simulink model "dsa2k_iwave_rfi"  (R2021a)
settings: Solver=VariableStepAuto  StartTime=0.0  StopTime=10.0  RelTol=1e-3
undefined symbols (not defined in the file): datetime, i, posixtime
libraries: xbsIndex_r4 x3053, casper_library_misc x61, rtr_casper_dsp_lib x31, xps_library x1
(part 1 of 43)
settings Model: Creator=jackh  LastModifiedBy=jackh

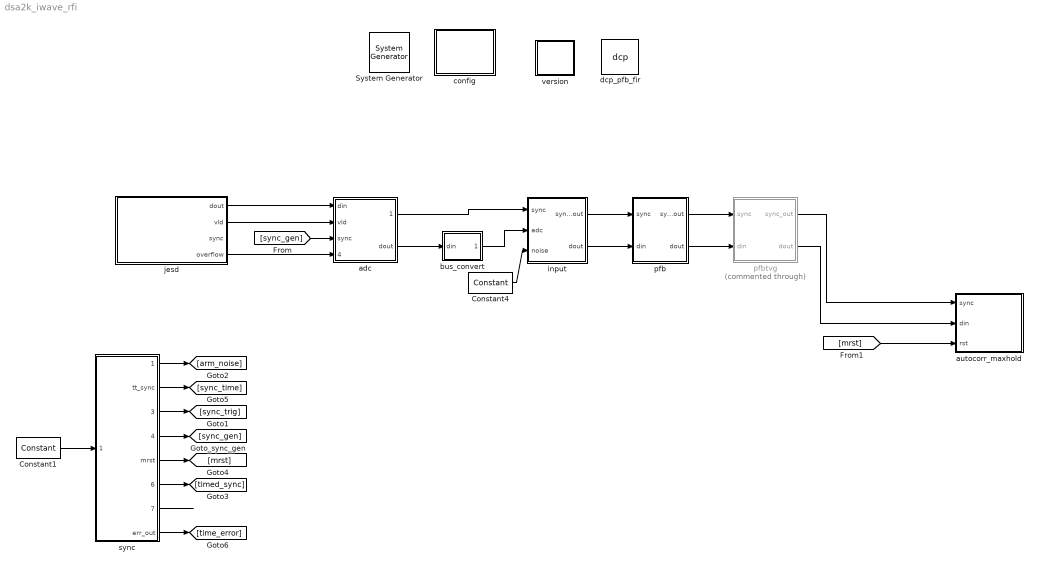
== system dsa2k_iwave_rfi ==
  " System Generator" : xbsIndex_r4/ System Generator  Tag=genX  xilinxfamily=zynquplus  part=xczu11eg  speed=-1-i  package=ffvc1760  synthesis_tool=XST  clock_wrapper=Clock Enables  directory=/home/jackh/src/dsa2000-fpga/firmware/src/models/dsa2k_iwave_rfi/sysgen  proj_type=Vivado  Synth_file=Vivado Synthesis Defaults  Impl_file=Vivado Implementation Defaults  testbench=off  simulink_period=1  sysclk_period=3.3333  dcm_input_clock_period=10  incr_netlist=off  trim_vbits=Everywhere in SubSystem  dbl_ovrd=According to Block Masks  core_generation=According to Block Masks  run_coregen=off  deprecated_control=off  eval_field=0  block_type=sysgen
  Constant1 : xbsIndex_r4/Constant  const=0  gui_display_data_type=Boolean  arith_type=Boolean  n_bits=16  bin_pt=14  preci_type=Single  exp_width=8  frac_width=24  explicit_period=on  period=1  equ=P=C  opselect=C  inp2=PCIN>>17  opr=+  inp1=P  carry=CIN  dbl_ovrd=off  block_type=constant
  Constant4 : xbsIndex_r4/Constant  const=0  gui_display_data_type=Fixed-point  arith_type=Unsigned  n_bits=12*32  bin_pt=0  preci_type=Single  exp_width=8  frac_width=24  explicit_period=on  period=1  equ=P=C  opselect=C  inp2=PCIN>>17  opr=+  inp1=P  carry=CIN  dbl_ovrd=off  block_type=constant
  adc : Subsystem  Tag=rtr:adc  AncestorBlock=rtr_casper_dsp_lib/adc  mask{ver_major=1, ver_minor=0, n_input=2, dtype='>i2'}
      mask prompts: ver_major "Block major version"; ver_minor "Block minor version"; n_input "Number of independent inputs"; dtype "Numpy sample data type"
  autocorr_maxhold : Subsystem  Tag=rtr:autocorr-maxhold  AncestorBlock=rtr_casper_dsp_lib/autocorr_maxhold  mask{rev_major=1, rev_minor=0, n_chan_serial_bits=14-3, n_chan_parallel_bits=3, n_input_serial_bits=0, n_input=2}
      mask prompts: rev_major "Major revision number"; rev_minor "Minor revision number"; n_chan_serial_bits "Number of *SERIAL* channels (2^?)"; n_chan_parallel_bits "Number of *PARALLEL* channels (2^?)"; n_input_serial_bits "Number of serial inputs (2^?)"; n_input "Total number of inputs"
  bus_convert : Subsystem  AncestorBlock=casper_library_bus/bus_convert  mask(bus_convert){n_bits_in=ones(32,1)*16, bin_pt_in=ones(32,1)*15, cmplx=off, n_bits_out=12, bin_pt_out=11, quantization=0, overflow=0, csp_latency=0, of=off, misc=off}
      mask prompts: n_bits_in "input bit widths"; bin_pt_in "input binary points"; cmplx "input complex"; n_bits_out "output bit widths"; bin_pt_out "output binary points"; quantization "quantization strategy (Truncate=0, Round  (unbiased: +/- Inf)=1, Round (unbiased: Even Values)=2)"; overflow "overflow strategy (Wrap=0, Saturate=1, Flag as error=2)"; csp_latency "latency"; of "overflow indication"; misc "misc support"
      mask help: Convert components of busses
      mask init:
      | bus_convert_init(gcb, ...
      |     'n_bits_in', n_bits_in, ...
      |     'bin_pt_in', bin_pt_in, ...
      |     'cmplx', cmplx, ...
      |     'n_bits_out', n_bits_out, ...
      |     'bin_pt_out', bin_pt_out, ...
      |     'quantization', quantization, ...
      |     'overflow', overflow, ...
      |     'csp_latency', csp_latency, ...
      |     'misc', misc, ...
      |     'of', of);
  config : Subsystem  Tag=xps:xsg  mask(xsg core config){hw_sys=iwave_zu11:xczu11eg, clk_src=adc_clk, clk_rate=4800/16, no_block_diagram=on, sample_period=1, synthesis_tool=XST}
      mask prompts: hw_sys "Hardware Platform"; clk_src "User IP Clock source"; clk_rate "User IP Clock Rate (MHz)"; no_block_diagram "Skip inclusion of infrastructure block diagram"; sample_period "Sample Period"; synthesis_tool "Synthesis Tool:"
      mask help:
      | The XSG Core Config block is used to configure the System Generator design
      | for the casper_xps toolflow. Settings here are used to configure the
      | Xilinx System Generator block parameters automatically, and control toolflow
      | script  execution. It needs to be at the top level of all designs being compiled
      | with the casper_xps toolflow.
      mask init:
      | xps_xsg_iwave_zu11_conf_mask;
      mask Help: eval('xlWeb([getenv(''MLIB_ROOT''), ''\doc\html\sys_xsg_core_config\sys_xsg_core_config.html''])')
      mask TypeOptions hw_sys: iwave_zu11:xczu11eg
      mask TypeOptions clk_src: sys_clk | adc_clk | clk300mhz
      mask TypeOptions synthesis_tool: Leonardo Spectrum | Synplify | Synplify Pro | XST
      mask Display: fprintf(['iWave_ZU11']);
  dcp_pfb_fir : xps_library/Utilities/dcp  Tag=xps:dcp  dcp_file=[fileparts(which(bdroot)) '/dsp/pfb_2p_32kpt_12i_18o_core/pfb_2p_32kpt_12i_18o_core.dcp']
      settings: SourceProductName=CASPER XPS Blockset
  input : Subsystem  Tag=rtr:input  AncestorBlock=rtr_casper_dsp_lib/input  mask{rev_major=1, rev_minor=0, n_bits=12, n_parallel=16, n_inputs=2}
      mask prompts: rev_major "Major revision number"; rev_minor "Minor revision number"; n_bits "Number of bits per samples"; n_parallel "Parallel Samples per input"; n_inputs "Parallel inputs"
  jesd : Subsystem  Tag=xps:adi_jesd  mask(xsg_adi_jesd){fmc_port=0, adi_ip_path=/home/jackh/src/dsa2000-fpga/firmware/lib/adi_hdl/library, sample_rate_mhz=4800}
      mask prompts: fmc_port "FMC Port Number"; adi_ip_path "Path to ADI IP repository"; sample_rate_mhz "Sample rate (Msps)"
      mask init:
      | adi_jesd_init()
      mask Help: eval('xlWeb([getenv(''MLIB_ROOT''), ''\doc\html\sys_xsg_core_config\sys_xsg_core_config.html''])')
  pfb : Subsystem  Tag=rtr:pfb  AncestorBlock=rtr_casper_dsp_lib/pfb  mask{rev_major=1, rev_minor=0, fft_bits=15}
      mask prompts: rev_major "Major revision number"; rev_minor "Minor revision number"; fft_bits "FFT length (2^?)"
  pfbtvg : Subsystem  Commented=through  mask{serial_chan_bits=14-3}
      mask prompts: serial_chan_bits "Serial channels (2^?)"
  sync : Subsystem  Tag=rtr:sync  AncestorBlock=rtr_casper_dsp_lib/sync  mask{rev_major=1, rev_minor=0, sync_lsb_bits=14, sync_period=12800000}
      mask prompts: rev_major "Rev Major"; rev_minor "Rev Minor"; sync_lsb_bits "Allowed sync granularity (2^?)"; sync_period "Expected_sync_period"
  version : Subsystem  Tag=rtr:version  AncestorBlock=rtr_casper_dsp_lib/version  mask{rev_major=1, rev_minor=0, fw_type=9, fw_ver_maj=1, fw_ver_min=0, fw_ver_rev=0, fw_ver_bugfix=0}
      mask prompts: rev_major "Rev Major (this block, not the firmware!)"; rev_minor "Rev Minor (this block, not the firmware!)"; fw_type "Firmware Type"; fw_ver_maj "Major version"; fw_ver_min "Minor version"; fw_ver_rev "Revision"; fw_ver_bugfix "Bugfix"
  wires:
  sync/1(arm_noise) -> [arm_noise]
  sync/2(tt_sync) -> [sync_time]
  sync/5(mrst) -> [mrst]
  sync/3(ext_sync) -> [sync_trig]
  sync/6(timed_sync) -> [timed_sync]
  sync/4(sync_out) -> [sync_gen]
  sync/8(err_out) -> [time_error]
  sync/7(tt_int_out) -> ?
  Constant1/1 -> sync/1(sync_in)
  adc/2(dout) -> bus_convert/1(din)
  pfbtvg/1(sync_out) -> autocorr_maxhold/1(sync)
  [mrst] -> autocorr_maxhold/3(rst)
  jesd/2(vld) -> adc/2(vld)
  jesd/4(overflow) -> adc/4(overflow)
  jesd/1(dout) -> adc/1(din)
  pfbtvg/2(dout) -> autocorr_maxhold/2(din)
  pfb/1(sync_out) -> pfbtvg/1(sync)
  pfb/2(dout) -> pfbtvg/2(din)
  [sync_gen] -> adc/3(sync)
  Constant4/1 -> input/3(noise)
  input/1(sync_out) -> pfb/1(sync)
  bus_convert/1(dout) -> input/2(adc)
  adc/1(sync_out) -> input/1(sync)
  input/2(dout) -> pfb/2(din)

== system dsa2k_iwave_rfi/adc ==
  din : Inport
  vld : Inport  Port=2
  sync : Inport  Port=3
  overflow : Inport  Port=4
  Inverter1 : xbsIndex_r4/Inverter  en=off  latency=1  dbl_ovrd=off  block_type=inv
  Logical : xbsIndex_r4/Logical  logical_function=OR  inputs=2  en=off  latency=0  precision=Full  arith_type=Unsigned  n_bits=16  bin_pt=0  align_bp=on  dbl_ovrd=off  block_type=logical
  Scope2 : Scope
  Scope3 : Scope
  Scope4 : Scope
  bitflip : Subsystem
  block_info : Subsystem  AncestorBlock=rtr_casper_dsp_lib/block_info
      mask init:
      | parent = get_param(gcb, 'Parent');
      | try
      |     params = get_param(parent, 'DialogParameters');
      | catch
      |     params = {};
      | end
      | info.library = 'rtr';
      | info.block_type = get_param(parent, 'Tag');
      | info.block_name = parent;
      | 
      | if length(params) > 0
      |     param_names = fieldnames(params);
      | else
      |     param_names = {};
      | end
      | n_param = length(param_names);
      | 
      | for n = 1:n_param
      |     param = param_names{n};
      |     val = get_param(parent, param);
      |     try
      |         val = eval(val);
      |     catch
      |     end
      |     info = setfield(info, param, val);
      | end
      | 
      | munge_block(gcb);
      | set_param([gcb '/info'], 'info', jsonencode(info));
  counter_led3 : xbsIndex_r4/Counter  cnt_type=Free Running  cnt_to=Inf  operation=Up  start_count=0  cnt_by_val=1  arith_type=Unsigned  n_bits=32  bin_pt=0  load_pin=off  rst=off  en=on  explicit_period=on  period=1  use_behavioral_HDL=off  implementation=Fabric  dbl_ovrd=off  block_type=counter
  counter_led4 : xbsIndex_r4/Counter  cnt_type=Free Running  cnt_to=Inf  operation=Up  start_count=0  cnt_by_val=1  arith_type=Unsigned  n_bits=32  bin_pt=0  load_pin=off  rst=off  en=on  explicit_period=on  period=1  use_behavioral_HDL=off  implementation=Fabric  dbl_ovrd=off  block_type=counter
  counter_led5 : xbsIndex_r4/Counter  cnt_type=Free Running  cnt_to=Inf  operation=Up  start_count=0  cnt_by_val=1  arith_type=Unsigned  n_bits=32  bin_pt=0  load_pin=off  rst=off  en=on  explicit_period=on  period=1  use_behavioral_HDL=off  implementation=Fabric  dbl_ovrd=off  block_type=counter
  edge_detect : casper_library_misc/edge_detect  edge=Rising  polarity=Active High  x_in=[0 0.08 0.08 0.16 0.16 0.24 0.24 0.32 0.32 0.4]  y_in="[-1 -1  1  1  1  1  1  1  1  1]"  x_out=[0.6 0.68 0.68 0.76 0.76 0.84 0.84 0.92 0.92 1]  y_out="[-1 -1  1  1 -1 -1 -1 -1 -1 -1]"
  edge_detect1 : casper_library_misc/edge_detect  edge=Rising  polarity=Active High  x_in=[0 0.08 0.08 0.16 0.16 0.24 0.24 0.32 0.32 0.4]  y_in="[-1 -1  1  1  1  1  1  1  1  1]"  x_out=[0.6 0.68 0.68 0.76 0.76 0.84 0.84 0.92 0.92 1]  y_out="[-1 -1  1  1 -1 -1 -1 -1 -1 -1]"
  invalid_counter : Subsystem  Tag=xps:sw_reg  AncestorBlock=xps_library/Memory/software_register  mask(swreg){io_dir=To Processor, io_delay=0, init_val=0, sample_period=1, names=reg, bitwidths=32, bin_pts=0, arith_types=0, sim_port=on, show_format=off}
      mask prompts: io_dir "I/O direction"; io_delay "I/O delay"; init_val "Initial Value"; sample_period "Sample period"; names "Bitfield names [msb...lsb]"; bitwidths "Bitfield widths"; bin_pts "Bitfield binary pts"; arith_types "Bitfield types, ufix=0, fix=1, bool=2"; sim_port "Provide sim input/output?"; show_format "Print format string?"
      mask help: A 32-bit software-accessible register. Can be divided into bitfields of varying widths and types using the fields in the block mask.
      mask init:
      | swreg_init(gcb)
      settings: AttributesFormatString=1output
      mask TypeOptions io_dir: To Processor | From Processor
      mask Callback io_dir:
      | mask_enables = get_param(gcb, 'MaskEnables');
      | mask_names = get_param(gcb, 'MaskNames');
      | if strcmp(get_param(gcb, 'io_dir'), 'To Processor'),
      |     mask_enables{ismember(mask_names, 'sample_period')} = 'off';
      | else
      |     mask_enables{ismember(mask_names, 'sample_period')} = 'on';
      | end
      | set_param(gcb, 'MaskEnables', mask_enables);
      mask DialogControl ParameterTabVar0 Prompt: Setup
  overflow_counter : Subsystem  Tag=xps:sw_reg  AncestorBlock=xps_library/Memory/software_register  mask(swreg){io_dir=To Processor, io_delay=0, init_val=0, sample_period=1, names=reg, bitwidths=32, bin_pts=0, arith_types=0, sim_port=on, show_format=off}
      mask prompts: io_dir "I/O direction"; io_delay "I/O delay"; init_val "Initial Value"; sample_period "Sample period"; names "Bitfield names [msb...lsb]"; bitwidths "Bitfield widths"; bin_pts "Bitfield binary pts"; arith_types "Bitfield types, ufix=0, fix=1, bool=2"; sim_port "Provide sim input/output?"; show_format "Print format string?"
      mask help: A 32-bit software-accessible register. Can be divided into bitfields of varying widths and types using the fields in the block mask.
      mask init:
      | swreg_init(gcb)
      settings: AttributesFormatString=1output
      mask TypeOptions io_dir: To Processor | From Processor
      mask Callback io_dir:
      | mask_enables = get_param(gcb, 'MaskEnables');
      | mask_names = get_param(gcb, 'MaskNames');
      | if strcmp(get_param(gcb, 'io_dir'), 'To Processor'),
      |     mask_enables{ismember(mask_names, 'sample_period')} = 'off';
      | else
      |     mask_enables{ismember(mask_names, 'sample_period')} = 'on';
      | end
      | set_param(gcb, 'MaskEnables', mask_enables);
      mask DialogControl ParameterTabVar0 Prompt: Setup
  snapshot_arm : Subsystem  Tag=xps:sw_reg  AncestorBlock=xps_library/Memory/software_register  mask(swreg){io_dir=From Processor, io_delay=0, init_val=0, sample_period=1, names=reg, bitwidths=1, bin_pts=0, arith_types=2, sim_port=on, show_format=off}
      mask prompts: io_dir "I/O direction"; io_delay "I/O delay"; init_val "Initial Value"; sample_period "Sample period"; names "Bitfield names [msb...lsb]"; bitwidths "Bitfield widths"; bin_pts "Bitfield binary pts"; arith_types "Bitfield types, ufix=0, fix=1, bool=2"; sim_port "Provide sim input/output?"; show_format "Print format string?"
      mask help: A 32-bit software-accessible register. Can be divided into bitfields of varying widths and types using the fields in the block mask.
      mask init:
      | swreg_init(gcb)
      settings: AttributesFormatString=1input
      mask TypeOptions io_dir: To Processor | From Processor
      mask Callback io_dir:
      | mask_enables = get_param(gcb, 'MaskEnables');
      | mask_names = get_param(gcb, 'MaskNames');
      | if strcmp(get_param(gcb, 'io_dir'), 'To Processor'),
      |     mask_enables{ismember(mask_names, 'sample_period')} = 'off';
      | else
      |     mask_enables{ismember(mask_names, 'sample_period')} = 'on';
      | end
      | set_param(gcb, 'MaskEnables', mask_enables);
      mask DialogControl ParameterTabVar0 Prompt: Setup
  snapshot_trig : Subsystem  Tag=xps:sw_reg  AncestorBlock=xps_library/Memory/software_register  mask(swreg){io_dir=From Processor, io_delay=0, init_val=0, sample_period=1, names=reg, bitwidths=1, bin_pts=0, arith_types=2, sim_port=on, show_format=off}
      mask prompts: io_dir "I/O direction"; io_delay "I/O delay"; init_val "Initial Value"; sample_period "Sample period"; names "Bitfield names [msb...lsb]"; bitwidths "Bitfield widths"; bin_pts "Bitfield binary pts"; arith_types "Bitfield types, ufix=0, fix=1, bool=2"; sim_port "Provide sim input/output?"; show_format "Print format string?"
      mask help: A 32-bit software-accessible register. Can be divided into bitfields of varying widths and types using the fields in the block mask.
      mask init:
      | swreg_init(gcb)
      settings: AttributesFormatString=1input
      mask TypeOptions io_dir: To Processor | From Processor
      mask Callback io_dir:
      | mask_enables = get_param(gcb, 'MaskEnables');
      | mask_names = get_param(gcb, 'MaskNames');
      | if strcmp(get_param(gcb, 'io_dir'), 'To Processor'),
      |     mask_enables{ismember(mask_names, 'sample_period')} = 'off';
      | else
      |     mask_enables{ismember(mask_names, 'sample_period')} = 'on';
      | end
      | set_param(gcb, 'MaskEnables', mask_enables);
      mask DialogControl ParameterTabVar0 Prompt: Setup
  ss : Subsystem
  sync_counter : Subsystem  Tag=xps:sw_reg  AncestorBlock=xps_library/Memory/software_register  mask(swreg){io_dir=To Processor, io_delay=0, init_val=0, sample_period=1, names=reg, bitwidths=32, bin_pts=0, arith_types=0, sim_port=on, show_format=off}
      mask prompts: io_dir "I/O direction"; io_delay "I/O delay"; init_val "Initial Value"; sample_period "Sample period"; names "Bitfield names [msb...lsb]"; bitwidths "Bitfield widths"; bin_pts "Bitfield binary pts"; arith_types "Bitfield types, ufix=0, fix=1, bool=2"; sim_port "Provide sim input/output?"; show_format "Print format string?"
      mask help: A 32-bit software-accessible register. Can be divided into bitfields of varying widths and types using the fields in the block mask.
      mask init:
      | swreg_init(gcb)
      settings: AttributesFormatString=1output
      mask TypeOptions io_dir: To Processor | From Processor
      mask Callback io_dir:
      | mask_enables = get_param(gcb, 'MaskEnables');
      | mask_names = get_param(gcb, 'MaskNames');
      | if strcmp(get_param(gcb, 'io_dir'), 'To Processor'),
      |     mask_enables{ismember(mask_names, 'sample_period')} = 'off';
      | else
      |     mask_enables{ismember(mask_names, 'sample_period')} = 'on';
      | end
      | set_param(gcb, 'MaskEnables', mask_enables);
      mask DialogControl ParameterTabVar0 Prompt: Setup
  sync_out : Outport
  dout : Outport  Port=2
  wires:
  Logical/1 -> ss/2(trig)
  Inverter1/1 -> counter_led5/1
  invalid_counter/1(sim_out_reg) -> Scope4/1
  counter_led5/1 -> invalid_counter/1(out_reg)
  vld/1 -> Inverter1/1, ss/1(we)
  counter_led4/1 -> sync_counter/1(out_reg)
  sync/1 -> Logical/1, counter_led4/1, sync_out/1
  edge_detect1/1 -> Logical/2
  sync_counter/1(sim_out_reg) -> Scope3/1
  snapshot_trig/1(in_reg) -> edge_detect1/1
  snapshot_arm/1(in_reg) -> edge_detect/1
  edge_detect/1 -> ss/3(arm)
  overflow_counter/1(sim_out_reg) -> Scope2/1
  counter_led3/1 -> overflow_counter/1(out_reg)
  overflow/1 -> counter_led3/1
  din/1 -> bitflip/1(bus_in)
  bitflip/1(bus_out) -> ss/4(bus_in), dout/1

== system dsa2k_iwave_rfi/autocorr_maxhold ==
  note: acc_len in spectra
  sync : Inport
  din : Inport  Port=2
  rst : Inport  Port=3
  0 : Subsystem  mask{nchan_bits=n_chan_serial_bits, npol_bits=n_input_serial_bits}
      mask prompts: nchan_bits "Number of channels (2^?)"; npol_bits "Number of pols (2^?)"
  1 : Subsystem  mask{nchan_bits=n_chan_serial_bits, npol_bits=n_input_serial_bits}
      mask prompts: nchan_bits "Number of channels (2^?)"; npol_bits "Number of pols (2^?)"
  Constant6 : Constant  Value=1024
  Counter1 : xbsIndex_r4/Counter  cnt_type=Free Running  cnt_to=Inf  operation=Up  start_count=0  cnt_by_val=1  arith_type=Unsigned  n_bits=32  bin_pt=0  load_pin=off  rst=off  en=on  explicit_period=on  period=1  use_behavioral_HDL=on  implementation=Fabric  dbl_ovrd=off  block_type=counter
  Delay1 : xbsIndex_r4/Delay  rst=off  infoeditControl=Selection of Reset will increase slice count due to use of real FFs and instead of SRLs  en=off  latency=1  reg_retiming=off  dbl_ovrd=off  block_type=delay
  Delay2 : xbsIndex_r4/Delay  rst=off  infoeditControl=Selection of Reset will increase slice count due to use of real FFs and instead of SRLs  en=off  latency=1  reg_retiming=on  dbl_ovrd=off  block_type=delay
  Slice1 : xbsIndex_r4/Slice  nbits=32 - n_chan_serial_bits - n_input_serial_bits  boolean_output=off  mode=Lower Bit Location + Width  bit1=0  base1=MSB of Input  bit0=0  base0=LSB of Input  dbl_ovrd=off  block_type=slice
  acc_cnt : Subsystem  Tag=xps:sw_reg  AncestorBlock=xps_library/Memory/software_register  mask(swreg){io_dir=To Processor, io_delay=0, init_val=0, sample_period=1, names=reg, bitwidths=32, bin_pts=0, arith_types=0, sim_port=on, show_format=on, desc_str=|}
      mask desc_str=|
      | 32-bit wrapping accumulation counter, which increments each
      | time a new accumulation is recorded to RAM.
      | There is no buffer locking when correlation data are
      | read, so this counter can be used to ensure that data
      | have not changed during a read.
      mask prompts: io_dir "I/O direction"; io_delay "I/O delay"; init_val "Initial Value"; sample_period "Sample period"; names "Bitfield names [msb...lsb]"; bitwidths "Bitfield widths"; bin_pts "Bitfield binary pts"; arith_types "Bitfield types, ufix=0, fix=1, bool=2"; sim_port "Provide sim input/output?"; show_format "Print format string?"; desc_str "Description"
      mask help: A 32-bit software-accessible register. Can be divided into bitfields of varying widths and types using the fields in the block mask.
      mask init:
      | swreg_init(gcb)
      settings: AttributesFormatString=1output:uf32.0 = 32 bits
      mask TypeOptions io_dir: To Processor | From Processor
      mask Callback io_dir:
      | mask_enables = get_param(gcb, 'MaskEnables');
      | mask_names = get_param(gcb, 'MaskNames');
      | if strcmp(get_param(gcb, 'io_dir'), 'To Processor'),
      |     mask_enables{ismember(mask_names, 'sample_period')} = 'off';
      | else
      |     mask_enables{ismember(mask_names, 'sample_period')} = 'on';
      | end
      | set_param(gcb, 'MaskEnables', mask_enables);
      mask DialogControl ParameterTabVar0 Prompt: Setup
  acc_len : Subsystem  Tag=xps:sw_reg  AncestorBlock=xps_library/Memory/software_register  mask(swreg){io_dir=From Processor, io_delay=0, init_val=0, sample_period=1, names=reg, bitwidths=32, bin_pts=0, arith_types=0, sim_port=on, show_format=on, desc_str=Accumulation length, in spectra.}
      mask prompts: io_dir "I/O direction"; io_delay "I/O delay"; init_val "Initial Value"; sample_period "Sample period"; names "Bitfield names [msb...lsb]"; bitwidths "Bitfield widths"; bin_pts "Bitfield binary pts"; arith_types "Bitfield types, ufix=0, fix=1, bool=2"; sim_port "Provide sim input/output?"; show_format "Print format string?"; desc_str "Description"
      mask help: A 32-bit software-accessible register. Can be divided into bitfields of varying widths and types using the fields in the block mask.
      mask init:
      | swreg_init(gcb)
      settings: AttributesFormatString=1input:uf32.0 = 32 bits
      mask TypeOptions io_dir: To Processor | From Processor
      mask Callback io_dir:
      | mask_enables = get_param(gcb, 'MaskEnables');
      | mask_names = get_param(gcb, 'MaskNames');
      | if strcmp(get_param(gcb, 'io_dir'), 'To Processor'),
      |     mask_enables{ismember(mask_names, 'sample_period')} = 'off';
      | else
      |     mask_enables{ismember(mask_names, 'sample_period')} = 'on';
      | end
      | set_param(gcb, 'MaskEnables', mask_enables);
      mask DialogControl ParameterTabVar0 Prompt: Setup
  block_info : Subsystem  AncestorBlock=rtr_casper_dsp_lib/block_info
      mask init: same as dsa2k_iwave_rfi/adc/block_info
  bus_expand : Subsystem  AncestorBlock=casper_library_flow_control/bus_expand  mask(bus_expand){mode=divisions of equal size, outputNum=2, outputWidth=36*8, outputBinaryPt=0, outputArithmeticType=0, show_format=off, outputToWorkspace=off, variablePrefix=out, outputToModelAsWell=on}
      mask prompts: outputNum "Number of outputs:"; outputWidth "Output width:"; outputBinaryPt "Output binary point position:"; outputArithmeticType "Output arithmetic type (ufix=0, fix=1, bool=2):"; show_format "Print format string?"; outputToWorkspace "Output to workspace?"; variablePrefix "Variable name prefix:"; outputToModelAsWell "Output to model as well?"
      mask help:
      | Expands a 'bus' made using a bus_create or Xilinx
      | concat block.
      | The input will be divided into the specified number
      | of outputs with the specified arithmetic types.
      | Divisions are made from most significant bit.
      mask init:
      | bus_expand_init(gcb,...
      |     'mode', mode, ...
      |     'outputNum', outputNum, ...
      |     'outputWidth', outputWidth, ...
      |     'outputBinaryPt', outputBinaryPt, ...
      |     'outputArithmeticType', outputArithmeticType, ...
      |     'show_format', show_format, ...
      |     'outputToWorkspace', outputToWorkspace, ...
      |     'variablePrefix', variablePrefix, ...
      |     'outputToModelAsWell', outputToModelAsWell);
      settings: AttributesFormatString=2 outputs
      mask TypeOptions mode: divisions of equal size | divisions of arbitrary size
      mask Callback mode: %bus_expand_callback();
      mask Callback outputWidth: %bus_expand_callback();
      mask Callback outputToWorkspace: %bus_expand_callback();
  trig : Subsystem  Tag=xps:sw_reg  AncestorBlock=xps_library/Memory/software_register  mask(swreg){io_dir=From Processor, io_delay=0, init_val=0, sample_period=1, names=reg, bitwidths=1, bin_pts=0, arith_types=2, sim_port=on, show_format=on, desc_str="Transition bit 0 from 0 to 1 to trigger a capture of the next valid accumulation"}
      mask prompts: io_dir "I/O direction"; io_delay "I/O delay"; init_val "Initial Value"; sample_period "Sample period"; names "Bitfield names [msb...lsb]"; bitwidths "Bitfield widths"; bin_pts "Bitfield binary pts"; arith_types "Bitfield types, ufix=0, fix=1, bool=2"; sim_port "Provide sim input/output?"; show_format "Print format string?"; desc_str "Description"
      mask help: A 32-bit software-accessible register. Can be divided into bitfields of varying widths and types using the fields in the block mask.
      mask init:
      | swreg_init(gcb)
      settings: AttributesFormatString=1input:b = 1 bits
      mask TypeOptions io_dir: To Processor | From Processor
      mask Callback io_dir:
      | mask_enables = get_param(gcb, 'MaskEnables');
      | mask_names = get_param(gcb, 'MaskNames');
      | if strcmp(get_param(gcb, 'io_dir'), 'To Processor'),
      |     mask_enables{ismember(mask_names, 'sample_period')} = 'off';
      | else
      |     mask_enables{ismember(mask_names, 'sample_period')} = 'on';
      | end
      | set_param(gcb, 'MaskEnables', mask_enables);
      mask DialogControl ParameterTabVar0 Prompt: Setup
  wires:
  Delay1/1 -> Counter1/1
  0/1(new_acc) -> [new_acc]
  [trig] -> 0/5(trig)
  trig/1(in_reg) -> [trig]
  [input0] -> 0/2(din)
  [acc_len] -> 0/4(acc_len)
  Counter1/1 -> Delay2/1
  Delay2/1 -> acc_cnt/1(out_reg)
  [new_acc] -> Delay1/1
  Slice1/1 -> [acc_len]
  Constant6/1 -> acc_len/1(sim_1)
  acc_len/1(in_reg) -> Slice1/1
  [rst] -> 0/3(rst)
  [sync] -> 0/1(sync)
  rst/1 -> [rst]
  sync/1 -> [sync]
  din/1 -> bus_expand/1(bus_in)
  bus_expand/1(msb_out2) -> [input0]
  bus_expand/2(lsb_out1) -> [input1]
  [sync] -> 1/1(sync)
  [rst] -> 1/3(rst)
  [acc_len] -> 1/4(acc_len)
  [input1] -> 1/2(din)
  [trig] -> 1/5(trig)

== system dsa2k_iwave_rfi/bus_convert ==
  din : Inport
  bussify : Subsystem  AncestorBlock=casper_library_flow_control/bus_create  mask(bus_create){inputNum=32}
      mask prompts: inputNum "Number of inputs:"
      mask init:
      | bus_create_init(gcb,...
      |     'inputNum', inputNum);
  conv{1..32} (32 alike) : xbsIndex_r4/Convert  gui_display_data_type=Fixed-point  arith_type="Signed  (2's comp)"  n_bits=12  bin_pt=11  float_type=Single  exp_bits=8  fraction_bits=24  quantization=Truncate  overflow=Wrap  en=off  latency=0  pipeline=on  dbl_ovrd=off  block_type=convert
  debus : Subsystem  AncestorBlock=casper_library_flow_control/bus_expand  mask(bus_expand){mode=divisions of arbitrary size, outputNum=2, outputWidth=[16;16;16;16;16;16;16;16;16;16;16;16;16;16;16;16;16;16;16;16;16;16;16;16;16;16;16;16;16;16;16;16], outputBinaryPt=[15;15;15;15;15;15;15;15;15;15;15;15;15;15;15;15;15;15;15;15;15;15;15;15;15;15;15;15;15;15;15;15], outputArithmeticType=[1 1 1 1 1 1 1 1 1 1 1 1 1 1 1 1 1 1 1 1 1 1 1 1 1 1 1 1 1 1 1 1], show_format=on, outputToWorkspace=off, variablePrefix=, outputToModelAsWell=on}
      mask prompts: outputNum "Number of outputs:"; outputWidth "Output width:"; outputBinaryPt "Output binary point position:"; outputArithmeticType "Output arithmetic type (ufix=0, fix=1, bool=2):"; show_format "Print format string?"; outputToWorkspace "Output to workspace?"; variablePrefix "Variable name prefix:"; outputToModelAsWell "Output to model as well?"
      mask help:
      | Expands a 'bus' made using a bus_create or Xilinx
      | concat block.
      | The input will be divided into the specified number
      | of outputs with the specified arithmetic types.
      | Divisions are made from most significant bit.
      mask init: same as dsa2k_iwave_rfi/autocorr_maxhold/bus_expand
      settings: AttributesFormatString=32 outputs: f16.15,f16.15,f16.15,f16.15,f16.15,f16.15,f16.15,f16.15,f16.15,f16.15,f16.15,f16.15,f16.15,f16.15,f16.15,f16.15,f16.15,f16.15,f16.15,f16.15,f16.15,f16.15,f16.15,f16.15,f16.15,f16.15,f16.15,f16.15,f16.15,f16.15,f16.15,f16.15,
      mask TypeOptions mode: divisions of equal size | divisions of arbitrary size
      mask Callback mode: %bus_expand_callback();
      mask Callback outputWidth: %bus_expand_callback();
      mask Callback outputToWorkspace: %bus_expand_callback();
  dout : Outport
  wires:
  din/1 -> debus/1(bus_in)
  debus/1(msb_out32) -> conv1/1
  debus/2(out31) -> conv2/1
  debus/3(out30) -> conv3/1
  debus/4(out29) -> conv4/1
  debus/5(out28) -> conv5/1
  debus/6(out27) -> conv6/1
  debus/7(out26) -> conv7/1
  debus/8(out25) -> conv8/1
  debus/9(out24) -> conv9/1
  debus/10(out23) -> conv10/1
  debus/11(out22) -> conv11/1
  debus/12(out21) -> conv12/1
  debus/13(out20) -> conv13/1
  debus/14(out19) -> conv14/1
  debus/15(out18) -> conv15/1
  debus/16(out17) -> conv16/1
  debus/17(out16) -> conv17/1
  debus/18(out15) -> conv18/1
  debus/19(out14) -> conv19/1
  debus/20(out13) -> conv20/1
  debus/21(out12) -> conv21/1
  debus/22(out11) -> conv22/1
  debus/23(out10) -> conv23/1
  debus/24(out9) -> conv24/1
  debus/25(out8) -> conv25/1
  debus/26(out7) -> conv26/1
  debus/27(out6) -> conv27/1
  debus/28(out5) -> conv28/1
  debus/29(out4) -> conv29/1
  debus/30(out3) -> conv30/1
  debus/31(out2) -> conv31/1
  debus/32(lsb_out1) -> conv32/1
  conv1/1 -> bussify/1(in1)
  conv2/1 -> bussify/2(in2)
  conv3/1 -> bussify/3(in3)
  conv4/1 -> bussify/4(in4)
  conv5/1 -> bussify/5(in5)
  conv6/1 -> bussify/6(in6)
  conv7/1 -> bussify/7(in7)
  conv8/1 -> bussify/8(in8)
  conv9/1 -> bussify/9(in9)
  conv10/1 -> bussify/10(in10)
  conv11/1 -> bussify/11(in11)
  conv12/1 -> bussify/12(in12)
  conv13/1 -> bussify/13(in13)
  conv14/1 -> bussify/14(in14)
  conv15/1 -> bussify/15(in15)
  conv16/1 -> bussify/16(in16)
  conv17/1 -> bussify/17(in17)
  conv18/1 -> bussify/18(in18)
  conv19/1 -> bussify/19(in19)
  conv20/1 -> bussify/20(in20)
  conv21/1 -> bussify/21(in21)
  conv22/1 -> bussify/22(in22)
  conv23/1 -> bussify/23(in23)
  conv24/1 -> bussify/24(in24)
  conv25/1 -> bussify/25(in25)
  conv26/1 -> bussify/26(in26)
  conv27/1 -> bussify/27(in27)
  conv28/1 -> bussify/28(in28)
  conv29/1 -> bussify/29(in29)
  conv30/1 -> bussify/30(in30)
  conv31/1 -> bussify/31(in31)
  conv32/1 -> bussify/32(in32)
  bussify/1(bus_out) -> dout/1

== system dsa2k_iwave_rfi/config ==

== system dsa2k_iwave_rfi/input ==
  sync : Inport
  adc : Inport  Port=2
  noise : Inport  Port=3
  Constant4 : xbsIndex_r4/Constant  const=0  gui_display_data_type=Fixed-point  arith_type=Unsigned  n_bits=n_bits * n_parallel * n_inputs  bin_pt=0  preci_type=Single  exp_width=8  frac_width=24  explicit_period=on  period=1  equ=P=C  opselect=C  inp2=PCIN>>17  opr=+  inp1=P  carry=CIN  dbl_ovrd=off  block_type=constant
  bit_stats : Subsystem  Commented=on
  block_info : Subsystem  AncestorBlock=rtr_casper_dsp_lib/block_info
      mask init: same as dsa2k_iwave_rfi/adc/block_info
  bus_mux1 : Subsystem  AncestorBlock=casper_library_bus/bus_mux  mask(bus_mux){n_inputs=3, n_bits=n_bits * n_parallel * ones(n_inputs,1), cmplx=off, misc=on, mux_latency=1}
      mask prompts: n_inputs "number of inputs"; n_bits "input bit widths"; cmplx "complex data"; misc "misc support"; mux_latency "mux latency"
      mask help: Mux components of bus
      mask init:
      | bus_mux_init(gcb, ...
      |     'n_inputs', n_inputs, ...
      |     'n_bits', n_bits, ...
      |     'cmplx', cmplx, ...
      |     'misc', misc, ...
      |     'mux_latency', mux_latency);
  rms : Subsystem
  slice3 : xbsIndex_r4/Slice  nbits=2*2  boolean_output=off  mode=Upper Bit Location + Width  bit1=0  base1=MSB of Input  bit0=0  base0=LSB of Input  dbl_ovrd=off  block_type=slice
  source_sel0 : Subsystem  Tag=xps:sw_reg  AncestorBlock=xps_library/Memory/software_register  mask(swreg){io_dir=From Processor, io_delay=0, init_val=0, sample_period=1, names=reg, bitwidths=32, bin_pts=0, arith_types=0, sim_port=on, show_format=off, desc_str=|}
      mask desc_str=|
      | Selector control to determine if signal streams carry
      | ADC samples, digital noise samples, or zeros.
      | Streams ``n=0..15`` is controlled by register
      | bits ``[2n+1:2n]``. Value ``0`` selects noise;
      | ``1`` selects ADC; ``2`` selects zeros.
      mask prompts: io_dir "I/O direction"; io_delay "I/O delay"; init_val "Initial Value"; sample_period "Sample period"; names "Bitfield names [msb...lsb]"; bitwidths "Bitfield widths"; bin_pts "Bitfield binary pts"; arith_types "Bitfield types, ufix=0, fix=1, bool=2"; sim_port "Provide sim input/output?"; show_format "Print format string?"; desc_str "Description"
      mask help: A 32-bit software-accessible register. Can be divided into bitfields of varying widths and types using the fields in the block mask.
      mask init:
      | swreg_init(gcb)
      settings: AttributesFormatString=1input
      mask TypeOptions io_dir: To Processor | From Processor
      mask Callback io_dir:
      | mask_enables = get_param(gcb, 'MaskEnables');
      | mask_names = get_param(gcb, 'MaskNames');
      | if strcmp(get_param(gcb, 'io_dir'), 'To Processor'),
      |     mask_enables{ismember(mask_names, 'sample_period')} = 'off';
      | else
      |     mask_enables{ismember(mask_names, 'sample_period')} = 'on';
      | end
      | set_param(gcb, 'MaskEnables', mask_enables);
      mask DialogControl ParameterTabVar0 Prompt: Setup
  sync_out : Outport  VectorParamsAs1DForOutWhenUnconnected=off
  dout : Outport  Port=2  VectorParamsAs1DForOutWhenUnconnected=off
  wires:
  sync/1 -> bus_mux1/5(misci)
  source_sel0/1(in_reg) -> slice3/1
  bus_mux1/2(misco) -> sync_out/1
  noise/1 -> bus_mux1/2(d0)
  adc/1 -> bus_mux1/3(d1)
  slice3/1 -> bus_mux1/1(sel)
  bus_mux1/1(out) -> dout/1, rms/1(in), bit_stats/1(din)
  Constant4/1 -> bus_mux1/4(d2)

== system dsa2k_iwave_rfi/jesd ==
  Convert : xbsIndex_r4/Convert  gui_display_data_type=Boolean  arith_type=Boolean  n_bits=16  bin_pt=14  float_type=Single  exp_bits=8  fraction_bits=24  quantization=Truncate  overflow=Wrap  en=off  latency=0  pipeline=off  dbl_ovrd=off  block_type=convert
  Convert1 : xbsIndex_r4/Convert  gui_display_data_type=Boolean  arith_type=Boolean  n_bits=16  bin_pt=14  float_type=Single  exp_bits=8  fraction_bits=24  quantization=Truncate  overflow=Wrap  en=off  latency=0  pipeline=off  dbl_ovrd=off  block_type=convert
  Convert2 : xbsIndex_r4/Convert  gui_display_data_type=Boolean  arith_type=Boolean  n_bits=16  bin_pt=14  float_type=Single  exp_bits=8  fraction_bits=24  quantization=Truncate  overflow=Wrap  en=off  latency=0  pipeline=off  dbl_ovrd=off  block_type=convert
  dsa2k_iwave_rfi_jesd_dout : xbsIndex_r4/Gateway In  gui_display_data_type=Fixed-point  arith_type=Unsigned  n_bits=512  bin_pt=0  preci_type=Single  exp_width=8  frac_width=24  rows=1  columns=1  quantization=Truncate  overflow=Wrap  period=1  UseAsADC=off  ADCChannel='1'  interface=None  automatic_assignment=on  address_offset=hex2dec('00')  intf_name=''  intf_description=''  default_value=0  timing_constraint=None  locs_specified=off  LOCs={}  io_standard={}  inherit_from_input=off  hdl_port=on  dbl_ovrd=off  block_type=gatewayin
  dsa2k_iwave_rfi_jesd_dout_overflow : xbsIndex_r4/Gateway In  gui_display_data_type=Fixed-point  arith_type=Unsigned  n_bits=1  bin_pt=0  preci_type=Single  exp_width=8  frac_width=24  rows=1  columns=1  quantization=Truncate  overflow=Wrap  period=1  UseAsADC=off  ADCChannel='1'  interface=None  automatic_assignment=on  address_offset=hex2dec('00')  intf_name=''  intf_description=''  default_value=0  timing_constraint=None  locs_specified=off  LOCs={}  io_standard={}  inherit_from_input=off  hdl_port=on  dbl_ovrd=off  block_type=gatewayin
  dsa2k_iwave_rfi_jesd_dout_sync : xbsIndex_r4/Gateway In  gui_display_data_type=Fixed-point  arith_type=Unsigned  n_bits=1  bin_pt=0  preci_type=Single  exp_width=8  frac_width=24  rows=1  columns=1  quantization=Truncate  overflow=Wrap  period=1  UseAsADC=off  ADCChannel='1'  interface=None  automatic_assignment=on  address_offset=hex2dec('00')  intf_name=''  intf_description=''  default_value=0  timing_constraint=None  locs_specified=off  LOCs={}  io_standard={}  inherit_from_input=off  hdl_port=on  dbl_ovrd=off  block_type=gatewayin
  dsa2k_iwave_rfi_jesd_dout_vld : xbsIndex_r4/Gateway In  gui_display_data_type=Fixed-point  arith_type=Unsigned  n_bits=1  bin_pt=0  preci_type=Single  exp_width=8  frac_width=24  rows=1  columns=1  quantization=Truncate  overflow=Wrap  period=1  UseAsADC=off  ADCChannel='1'  interface=None  automatic_assignment=on  address_offset=hex2dec('00')  intf_name=''  intf_description=''  default_value=0  timing_constraint=None  locs_specified=off  LOCs={}  io_standard={}  inherit_from_input=off  hdl_port=on  dbl_ovrd=off  block_type=gatewayin
  dout : Outport  VectorParamsAs1DForOutWhenUnconnected=off
  vld : Outport  Port=2  VectorParamsAs1DForOutWhenUnconnected=off
  sync : Outport  Port=3  VectorParamsAs1DForOutWhenUnconnected=off
  overflow : Outport  Port=4  VectorParamsAs1DForOutWhenUnconnected=off
  wires:
  dsa2k_iwave_rfi_jesd_dout/1 -> dout/1
  dsa2k_iwave_rfi_jesd_dout_vld/1 -> Convert/1
  dsa2k_iwave_rfi_jesd_dout_sync/1 -> Convert1/1
  dsa2k_iwave_rfi_jesd_dout_overflow/1 -> Convert2/1
  Convert/1 -> vld/1
  Convert1/1 -> sync/1
  Convert2/1 -> overflow/1

== system dsa2k_iwave_rfi/pfb ==
  sync : Inport
  din : Inport  Port=2
  Black Box : xbsIndex_r4/Black Box  init_code=pfb_2p_32kpt_12i_18o_core_config  sim_method=ISE Simulator  verbose=off  block_type=blackbox2
  Counter : xbsIndex_r4/Counter  cnt_type=Free Running  cnt_to=Inf  operation=Up  start_count=0  cnt_by_val=1  arith_type=Unsigned  n_bits=32  bin_pt=0  load_pin=off  rst=on  en=on  explicit_period=on  period=1  use_behavioral_HDL=on  implementation=DSP48  dbl_ovrd=off  block_type=counter
  block_info : Subsystem  AncestorBlock=rtr_casper_dsp_lib/block_info
      mask init: same as dsa2k_iwave_rfi/adc/block_info
  bus_create : Subsystem  AncestorBlock=casper_library_flow_control/bus_create  mask(bus_create){inputNum=2}
      mask prompts: inputNum "Number of inputs:"
      mask init:
      | bus_create_init(gcb,...
      |     'inputNum', inputNum);
  bus_expand : Subsystem  AncestorBlock=casper_library_flow_control/bus_expand  mask(bus_expand){mode=divisions of equal size, outputNum=2, outputWidth=12*16, outputBinaryPt=0, outputArithmeticType=0, show_format=off, outputToWorkspace=off, variablePrefix=out, outputToModelAsWell=on}
      mask prompts: outputNum "Number of outputs:"; outputWidth "Output width:"; outputBinaryPt "Output binary point position:"; outputArithmeticType "Output arithmetic type (ufix=0, fix=1, bool=2):"; show_format "Print format string?"; outputToWorkspace "Output to workspace?"; variablePrefix "Variable name prefix:"; outputToModelAsWell "Output to model as well?"
      mask help:
      | Expands a 'bus' made using a bus_create or Xilinx
      | concat block.
      | The input will be divided into the specified number
      | of outputs with the specified arithmetic types.
      | Divisions are made from most significant bit.
      mask init: same as dsa2k_iwave_rfi/autocorr_maxhold/bus_expand
      settings: AttributesFormatString=2 outputs
      mask TypeOptions mode: divisions of equal size | divisions of arbitrary size
      mask Callback mode: %bus_expand_callback();
      mask Callback outputWidth: %bus_expand_callback();
      mask Callback outputToWorkspace: %bus_expand_callback();
  ctrl : Subsystem  Tag=xps:sw_reg  AncestorBlock=xps_library/Memory/software_register  mask(swreg){io_dir=From Processor, io_delay=0, init_val=0, sample_period=1, names=reg, bitwidths=1, bin_pts=0, arith_types=2, sim_port=on, show_format=on, desc_str=""}
      mask prompts: io_dir "I/O direction"; io_delay "I/O delay"; init_val "Initial Value"; sample_period "Sample period"; names "Bitfield names [msb...lsb]"; bitwidths "Bitfield widths"; bin_pts "Bitfield binary pts"; arith_types "Bitfield types, ufix=0, fix=1, bool=2"; sim_port "Provide sim input/output?"; show_format "Print format string?"; desc_str "Description"
      mask help: A 32-bit software-accessible register. Can be divided into bitfields of varying widths and types using the fields in the block mask.
      mask init:
      | swreg_init(gcb)
      settings: AttributesFormatString=1input:b = 1 bits
      mask TypeOptions io_dir: To Processor | From Processor
      mask Callback io_dir:
      | mask_enables = get_param(gcb, 'MaskEnables');
      | mask_names = get_param(gcb, 'MaskNames');
      | if strcmp(get_param(gcb, 'io_dir'), 'To Processor'),
      |     mask_enables{ismember(mask_names, 'sample_period')} = 'off';
      | else
      |     mask_enables{ismember(mask_names, 'sample_period')} = 'on';
      | end
      | set_param(gcb, 'MaskEnables', mask_enables);
      mask DialogControl ParameterTabVar0 Prompt: Setup
  of_count : Subsystem  Tag=xps:sw_reg  AncestorBlock=xps_library/Memory/software_register  mask(swreg){io_dir=To Processor, io_delay=0, init_val=0, sample_period=1, names=reg, bitwidths=32, bin_pts=0, arith_types=0, sim_port=on, show_format=on, desc_str=""}
      mask prompts: io_dir "I/O direction"; io_delay "I/O delay"; init_val "Initial Value"; sample_period "Sample period"; names "Bitfield names [msb...lsb]"; bitwidths "Bitfield widths"; bin_pts "Bitfield binary pts"; arith_types "Bitfield types, ufix=0, fix=1, bool=2"; sim_port "Provide sim input/output?"; show_format "Print format string?"; desc_str "Description"
      mask help: A 32-bit software-accessible register. Can be divided into bitfields of varying widths and types using the fields in the block mask.
      mask init:
      | swreg_init(gcb)
      settings: AttributesFormatString=1output:uf32.0 = 32 bits
      mask TypeOptions io_dir: To Processor | From Processor
      mask Callback io_dir:
      | mask_enables = get_param(gcb, 'MaskEnables');
      | mask_names = get_param(gcb, 'MaskNames');
      | if strcmp(get_param(gcb, 'io_dir'), 'To Processor'),
      |     mask_enables{ismember(mask_names, 'sample_period')} = 'off';
      | else
      |     mask_enables{ismember(mask_names, 'sample_period')} = 'on';
      | end
      | set_param(gcb, 'MaskEnables', mask_enables);
      mask DialogControl ParameterTabVar0 Prompt: Setup
  shift : Subsystem  Tag=xps:sw_reg  AncestorBlock=xps_library/Memory/software_register  mask(swreg){io_dir=From Processor, io_delay=0, init_val=0, sample_period=1, names=reg, bitwidths=32, bin_pts=0, arith_types=0, sim_port=on, show_format=on, desc_str=""}
      mask prompts: io_dir "I/O direction"; io_delay "I/O delay"; init_val "Initial Value"; sample_period "Sample period"; names "Bitfield names [msb...lsb]"; bitwidths "Bitfield widths"; bin_pts "Bitfield binary pts"; arith_types "Bitfield types, ufix=0, fix=1, bool=2"; sim_port "Provide sim input/output?"; show_format "Print format string?"; desc_str "Description"
      mask help: A 32-bit software-accessible register. Can be divided into bitfields of varying widths and types using the fields in the block mask.
      mask init:
      | swreg_init(gcb)
      settings: AttributesFormatString=1input:uf32.0 = 32 bits
      mask TypeOptions io_dir: To Processor | From Processor
      mask Callback io_dir:
      | mask_enables = get_param(gcb, 'MaskEnables');
      | mask_names = get_param(gcb, 'MaskNames');
      | if strcmp(get_param(gcb, 'io_dir'), 'To Processor'),
      |     mask_enables{ismember(mask_names, 'sample_period')} = 'off';
      | else
      |     mask_enables{ismember(mask_names, 'sample_period')} = 'on';
      | end
      | set_param(gcb, 'MaskEnables', mask_enables);
      mask DialogControl ParameterTabVar0 Prompt: Setup
  sync_out : Outport  VectorParamsAs1DForOutWhenUnconnected=off
  dout : Outport  Port=2  VectorParamsAs1DForOutWhenUnconnected=off
  wires:
  Black Box/4 -> Counter/2
  [stat_rst] -> Counter/1
  ctrl/1(in_reg) -> [stat_rst]
  Black Box/3 -> bus_create/2(in2)
  Black Box/2 -> bus_create/1(in1)
  Black Box/1 -> sync_out/1
  sync/1 -> Black Box/1
  Counter/1 -> of_count/1(out_reg)
  shift/1(in_reg) -> Black Box/2
  bus_create/1(bus_out) -> dout/1
  bus_expand/2(lsb_out1) -> Black Box/4
  bus_expand/1(msb_out2) -> Black Box/3
  din/1 -> bus_expand/1(bus_in)

== system dsa2k_iwave_rfi/pfbtvg ==
  sync : Inport
  din : Inport  Port=2
  0 : Subsystem
  Delay1 : xbsIndex_r4/Delay  rst=off  infoeditControl=Selection of Reset will increase slice count due to use of real FFs and instead of SRLs  en=off  latency=1  reg_retiming=on  dbl_ovrd=off  block_type=delay
  Delay2 : xbsIndex_r4/Delay  rst=off  infoeditControl=Selection of Reset will increase slice count due to use of real FFs and instead of SRLs  en=off  latency=1  reg_retiming=on  dbl_ovrd=off  block_type=delay
  Delay3 : xbsIndex_r4/Delay  rst=off  infoeditControl=Selection of Reset will increase slice count due to use of real FFs and instead of SRLs  en=off  latency=1  reg_retiming=on  dbl_ovrd=off  block_type=delay
  Mux : xbsIndex_r4/Mux  inputs=2  en=off  latency=1  precision=Full  arith_type=Unsigned  n_bits=16  bin_pt=14  quantization=Truncate  overflow=Wrap  dbl_ovrd=off  block_type=mux
  ctrl : Subsystem  Tag=xps:sw_reg  AncestorBlock=xps_library/Memory/software_register  mask(swreg){io_dir=From Processor, io_delay=0, init_val=0, sample_period=1, names=reg, bitwidths=1, bin_pts=0, arith_types=2, sim_port=on, show_format=on, desc_str=""}
      mask prompts: io_dir "I/O direction"; io_delay "I/O delay"; init_val "Initial Value"; sample_period "Sample period"; names "Bitfield names [msb...lsb]"; bitwidths "Bitfield widths"; bin_pts "Bitfield binary pts"; arith_types "Bitfield types, ufix=0, fix=1, bool=2"; sim_port "Provide sim input/output?"; show_format "Print format string?"; desc_str "Description"
      mask help: A 32-bit software-accessible register. Can be divided into bitfields of varying widths and types using the fields in the block mask.
      mask init:
      | swreg_init(gcb)
      settings: AttributesFormatString=1input:b = 1 bits
      mask TypeOptions io_dir: To Processor | From Processor
      mask Callback io_dir:
      | mask_enables = get_param(gcb, 'MaskEnables');
      | mask_names = get_param(gcb, 'MaskNames');
      | if strcmp(get_param(gcb, 'io_dir'), 'To Processor'),
      |     mask_enables{ismember(mask_names, 'sample_period')} = 'off';
      | else
      |     mask_enables{ismember(mask_names, 'sample_period')} = 'on';
      | end
      | set_param(gcb, 'MaskEnables', mask_enables);
      mask DialogControl ParameterTabVar0 Prompt: Setup
  sync_out : Outport  VectorParamsAs1DForOutWhenUnconnected=off
  dout : Outport  Port=2  VectorParamsAs1DForOutWhenUnconnected=off
  wires:
  sync/1 -> 0/1(rst), Delay2/1
  Mux/1 -> dout/1
  ctrl/1(in_reg) -> [tvg_en]
  Delay2/1 -> Delay3/1
  0/1(dout) -> Mux/3
  [tvg_en] -> Mux/1
  Delay3/1 -> sync_out/1
  din/1 -> Delay1/1
  Delay1/1 -> Mux/2
